simulink model "fuzzypid"  (R2018b)
settings: Solver=VariableStepAuto  StartTime=0.0  StopTime=10.0  RelTol=1e-3
libraries: fuzblock x1
settings Model: Creator=nila  LastModifiedBy=root
settings SFSimCC: SimUseLocalCustomCode=off
settings RTWCC: RTWUseLocalCustomCode=off
settings CodeAppCC: StateflowObjectComments=on

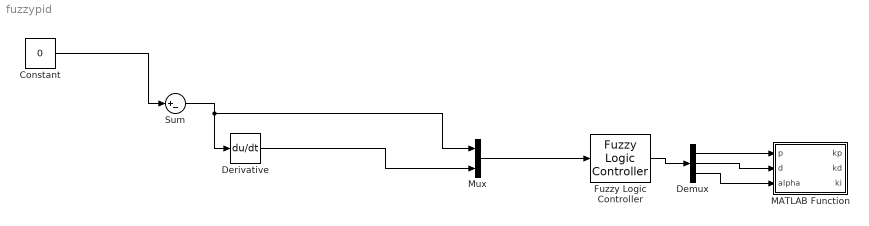
== system fuzzypid ==
  Constant : Constant  Value=0
  Demux : Demux  Outputs=3
  Derivative : Derivative
  Fuzzy Logic Controller : fuzblock/Fuzzy Logic  Controller  FIS=fuzzypid.fis  OutputSampleNumber=101  DataType=double  FuzzifiedInputs=off  RuleFiringStrengths=off  RuleOutputs=off  AggregatedOutputs=off  SimulateUsing=Interpreted execution  OutOfRangeInputValueMessage=warning  NoRuleFiredMessage=warning  EmptyOutputFuzzySetMessage=warning
  MATLAB Function : MATLAB Function  TreatAsAtomicUnit=on
  Mux : Mux  Inputs=2
  Sum : Sum  Inputs=|+-
  wires:
  Constant/1 -> Sum/1
  Mux/1 -> Fuzzy Logic Controller/1
  Sum/1 -> Mux/1, Derivative/1
  Derivative/1 -> Mux/2
  Fuzzy Logic Controller/1 -> Demux/1
  Demux/1 -> MATLAB Function/1(p)
  Demux/2 -> MATLAB Function/2(d)
  Demux/3 -> MATLAB Function/3(alpha)

== matlab function fuzzypid/MATLAB Function ==
  data: p input; d input; kp output; alpha input; kd output; ki output
function [kp, kd, ki] =  fuzzypid(p, d, alpha)
kpmin=0;
kpmax=0;
kdmin=0;
kdmax=0;
kp = p*(kpmax - kpmin) + kpmin ;
kd = d*(kdmax - kdmin) + kdmin ;
ki = kd/alpha ;
end
